simulink model "MagneticLevitator"  (R2025b)
settings: Solver=VariableStepAuto  StartTime=0.0  StopTime=1.0  RelTol=1e-3
undefined symbols (not defined in the file): g, K_force, L, m, R, R_coil, Vsup, x0
settings Model: Creator=lucianbracy  LastModifiedBy=lucianbracy

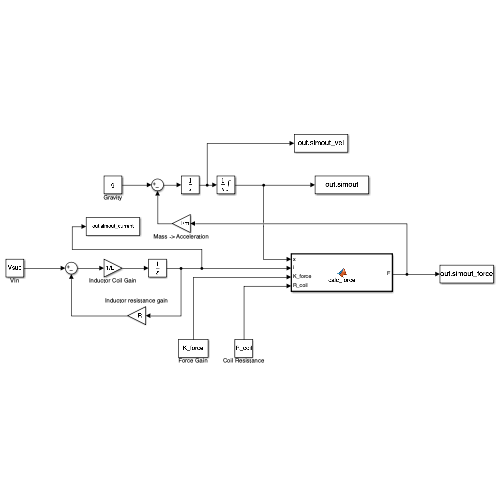
[thumbnail: Simulink's stored preview of the top-level diagram]
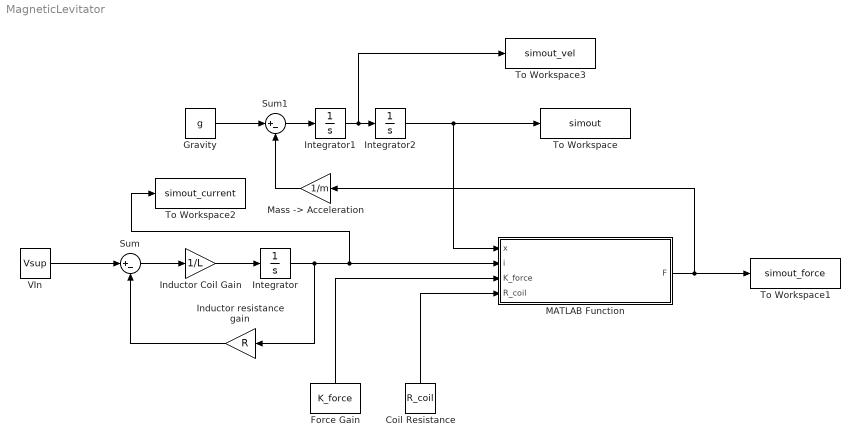
== system MagneticLevitator ==
  Coil Resistance : Constant  Value=R_coil
  Force Gain : Constant  Value=K_force
  Gravity : Constant  Value=g
  Inductor Coil Gain : Gain  Gain=1/L
  Inductor resistance gain : Gain  Gain=R
  Integrator : Integrator
  Integrator1 : Integrator
  Integrator2 : Integrator  InitialCondition=x0  LimitOutput=on  UpperSaturationLimit=0.0254  LowerSaturationLimit=0.000001
  MATLAB Function : MATLAB Function  TreatAsAtomicUnit=on
  "Mass -> Acceleration" : Gain  Gain=1/m
  Sum : Sum  Inputs=|+-
  Sum1 : Sum  Inputs=|+-
  To Workspace : ToWorkspace  VariableName=simout  SaveFormat=Timeseries  SampleTime=-1
  To Workspace1 : ToWorkspace  VariableName=simout_force  SaveFormat=Timeseries  SampleTime=-1
  To Workspace2 : ToWorkspace  VariableName=simout_current  SaveFormat=Timeseries  SampleTime=-1
  To Workspace3 : ToWorkspace  VariableName=simout_vel  SaveFormat=Timeseries  SampleTime=-1
  VIn : Constant  Value=Vsup
  wires:
  VIn/1 -> Sum/1
  Sum/1 -> Inductor Coil Gain/1
  Inductor Coil Gain/1 -> Integrator/1
  Inductor resistance gain/1 -> Sum/2
  Integrator/1 -> To Workspace2/1, MATLAB Function/2(i), Inductor resistance gain/1
  Force Gain/1 -> MATLAB Function/3(K_force)
  Coil Resistance/1 -> MATLAB Function/4(R_coil)
  Gravity/1 -> Sum1/1
  MATLAB Function/1(F) -> To Workspace1/1, "Mass -> Acceleration"/1
  "Mass -> Acceleration"/1 -> Sum1/2
  Sum1/1 -> Integrator1/1
  Integrator1/1 -> To Workspace3/1, Integrator2/1
  Integrator2/1 -> To Workspace/1, MATLAB Function/1(x)

== matlab function MagneticLevitator/MATLAB Function ==
  data: x input; F output; i input; K_force input; R_coil input
function F = calc_force(x, i, K_force, R_coil)
    F = K_force * (i * x) / (x^2 + R_coil^2)^2.5;
end
